simulink model "compare_pst_kapa_tau"  (R2020b)
settings: Solver=FixedStepAuto  StartTime=0.0  StopTime=250  FixedStep=t0  RelTol=1e-3
undefined symbols (not defined in the file or in its folder): P_kap, P_tau, plant_1, S_kap, S_tau, t0, T_kap, T_tau
settings Model: Creator=user1  LastModifiedBy=rafael
settings SFSimCC: CustomCodeUndefinedFunction=UseInterfaceOnly

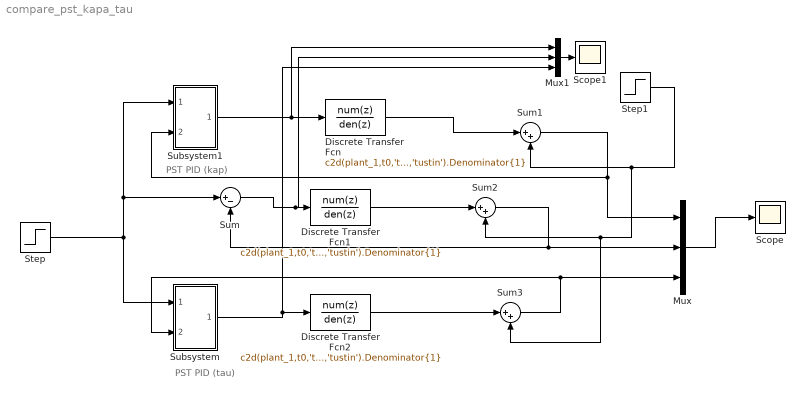
== system compare_pst_kapa_tau ==
  note: PST PID (kap)
  note: PST PID (tau)
  Discrete Transfer Fcn : DiscreteTransferFcn  Numerator=c2d(plant_1,t0,'tustin').Numerator{1}  Denominator=c2d(plant_1,t0,'tustin').Denominator{1}  SampleTime=t0
  Discrete Transfer Fcn1 : DiscreteTransferFcn  Numerator=c2d(plant_1,t0,'tustin').Numerator{1}  Denominator=c2d(plant_1,t0,'tustin').Denominator{1}  SampleTime=t0
  Discrete Transfer Fcn2 : DiscreteTransferFcn  Numerator=c2d(plant_1,t0,'tustin').Numerator{1}  Denominator=c2d(plant_1,t0,'tustin').Denominator{1}  SampleTime=t0
  Mux : Mux  Inputs=3
  Mux1 : Mux  Inputs=3
  Scope : Scope
  Scope1 : Scope
  Step : Step  SampleTime=0
  Step1 : Step  Time=100  SampleTime=0
  Subsystem : Subsystem
  Subsystem1 : Subsystem
  Sum : Sum  Inputs=|+-
  Sum1 : Sum  Inputs=|++
  Sum2 : Sum  Inputs=|++
  Sum3 : Sum  Inputs=|++
  wires:
  Step/1 -> Subsystem1/1(In1), Sum/1, Subsystem/1(In1)
  Subsystem/1(Out1) -> Discrete Transfer Fcn2/1, Mux1/3
  Mux/1 -> Scope/1
  Sum/1 -> Mux1/2, Discrete Transfer Fcn1/1
  Subsystem1/1(Out1) -> Discrete Transfer Fcn/1, Mux1/1
  Mux1/1 -> Scope1/1
  Step1/1 -> Sum3/2, Sum2/2, Sum1/2
  Discrete Transfer Fcn/1 -> Sum1/1
  Sum1/1 -> Mux/1, Subsystem1/2(In2)
  Discrete Transfer Fcn2/1 -> Sum3/1
  Discrete Transfer Fcn1/1 -> Sum2/1
  Sum3/1 -> Subsystem/2(In2), Mux/3
  Sum2/1 -> Mux/2, Sum/2

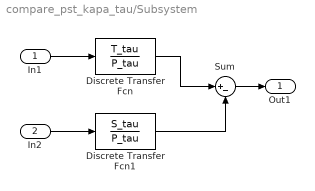
== system compare_pst_kapa_tau/Subsystem ==
  In1 : Inport
  In2 : Inport  Port=2
  Discrete Transfer Fcn : DiscreteTransferFcn  Numerator=T_tau  Denominator=P_tau
  Discrete Transfer Fcn1 : DiscreteTransferFcn  Numerator=S_tau  Denominator=P_tau
  Sum : Sum  Inputs=|+-
  Out1 : Outport  VectorParamsAs1DForOutWhenUnconnected=off
  wires:
  In2/1 -> Discrete Transfer Fcn1/1
  Discrete Transfer Fcn1/1 -> Sum/2
  Sum/1 -> Out1/1
  Discrete Transfer Fcn/1 -> Sum/1
  In1/1 -> Discrete Transfer Fcn/1

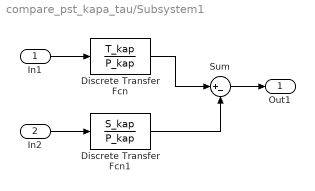
== system compare_pst_kapa_tau/Subsystem1 ==
  In1 : Inport
  In2 : Inport  Port=2
  Discrete Transfer Fcn : DiscreteTransferFcn  Numerator=T_kap  Denominator=P_kap  SampleTime=t0
  Discrete Transfer Fcn1 : DiscreteTransferFcn  Numerator=S_kap  Denominator=P_kap  SampleTime=t0
  Sum : Sum  Inputs=|+-
  Out1 : Outport  VectorParamsAs1DForOutWhenUnconnected=off
  wires:
  In1/1 -> Discrete Transfer Fcn/1
  In2/1 -> Discrete Transfer Fcn1/1
  Discrete Transfer Fcn/1 -> Sum/1
  Discrete Transfer Fcn1/1 -> Sum/2
  Sum/1 -> Out1/1
